simulink library "packLibrary"  (R2022b)
settings: Solver=VariableStepAuto  StartTime=0.0  StopTime=10.0  RelTol=1e-3
undefined symbols (not defined in the file): battery_builder_rtmsupport, gcbh
libraries: packLibrary_lib x12
settings Model: Creator=DELL  LastModifiedBy=DELL

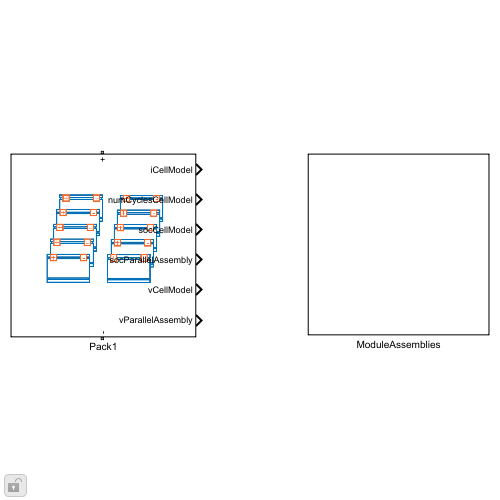
[thumbnail: Simulink's stored preview of the top-level diagram]
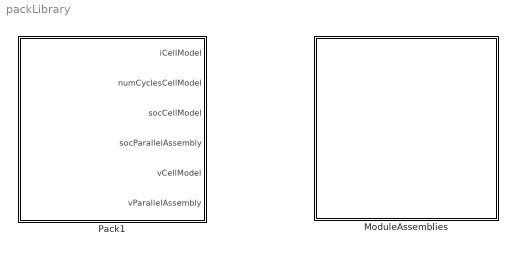
== system packLibrary ==
  ModuleAssemblies : Subsystem
  Pack1 : Subsystem  LoadFcn=battery_builder_rtmsupport('loadfcn',gcbh);
      settings: CopyFcn=battery_builder_rtmsupport('copyfcn',gcbh);  PreCopyFcn=battery_builder_rtmsupport('precopyfcn',gcbh);  PreDeleteFcn=battery_builder_rtmsupport('predeletefcn',gcbh);  PortSchema="{\"entries\":[{\"content\":{\"sides\":[{\"content\":{\"connectorIds\":[\"LConn1\"]},\"type\":\"ConnectorPlacement.EquallySpacedRectSide\",\"uuid\":\"28c6eb33-4d49-4fb1-9cde-b9dfdd77c876\"},{\"content\":{\"connectorIds\":[\"RConn1\"],\"side\":\"RIGHT\"},\"type\":\"ConnectorPlacement.EquallySpacedRectSide\",\"uuid\":\"b9810162-5634-4adf-aff8-c39045d02da2\"},{\"content\":{\"connectorIds\":[],\"side\":\"TOP\"},\"type\":\"ConnectorPlacement.EquallySpacedRectSide\",\"uuid\":\"1ba0f325-5e56-4337-925f-22d4ca88eb4a\"},{\"content\":{\"connectorIds\":[\"Out1\",\"Out2\",\"Out3\",\"Out4\",\"Out5\",\"Out6\"],\"side\":\"BOTTOM\"},\"type\":\"ConnectorPlacement.EquallySpacedRectSide\",\"uuid\":\"96c4fc69-b9f6-473b-8733-ab7f3394c566\"}]},\"type\":\"ConnectorPlacement.EquallySpacedConnector\",\"uuid\":\"e67f4e04-d31b-4901-b860-df486ab909d4\"}],\"packageUris\":[\"http://schema.mathworks.com/mf0/Connector/R2020b\"],\"version\":\"1.0\"}"
      mask Display: image('$imagefile')

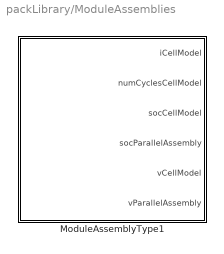
== system packLibrary/ModuleAssemblies ==
  ModuleAssemblyType1 : Subsystem  LoadFcn=battery_builder_rtmsupport('loadfcn',gcbh);
      settings: CopyFcn=battery_builder_rtmsupport('copyfcn',gcbh);  PreCopyFcn=battery_builder_rtmsupport('precopyfcn',gcbh);  PreDeleteFcn=battery_builder_rtmsupport('predeletefcn',gcbh);  PortSchema="{\"entries\":[{\"content\":{\"sides\":[{\"content\":{\"connectorIds\":[\"LConn1\"]},\"type\":\"ConnectorPlacement.EquallySpacedRectSide\",\"uuid\":\"28c6eb33-4d49-4fb1-9cde-b9dfdd77c876\"},{\"content\":{\"connectorIds\":[\"RConn1\"],\"side\":\"RIGHT\"},\"type\":\"ConnectorPlacement.EquallySpacedRectSide\",\"uuid\":\"b9810162-5634-4adf-aff8-c39045d02da2\"},{\"content\":{\"connectorIds\":[],\"side\":\"TOP\"},\"type\":\"ConnectorPlacement.EquallySpacedRectSide\",\"uuid\":\"1ba0f325-5e56-4337-925f-22d4ca88eb4a\"},{\"content\":{\"connectorIds\":[\"Out1\",\"Out2\",\"Out3\",\"Out4\",\"Out5\",\"Out6\"],\"side\":\"BOTTOM\"},\"type\":\"ConnectorPlacement.EquallySpacedRectSide\",\"uuid\":\"d11a51c6-486f-4741-a229-6ae1ae8804c6\"}]},\"type\":\"ConnectorPlacement.EquallySpacedConnector\",\"uuid\":\"e67f4e04-d31b-4901-b860-df486ab909d4\"}],\"packageUris\":[\"http://schema.mathworks.com/mf0/Connector/R2020b\"],\"version\":\"1.0\"}"
      mask Display: image('$imagefile')

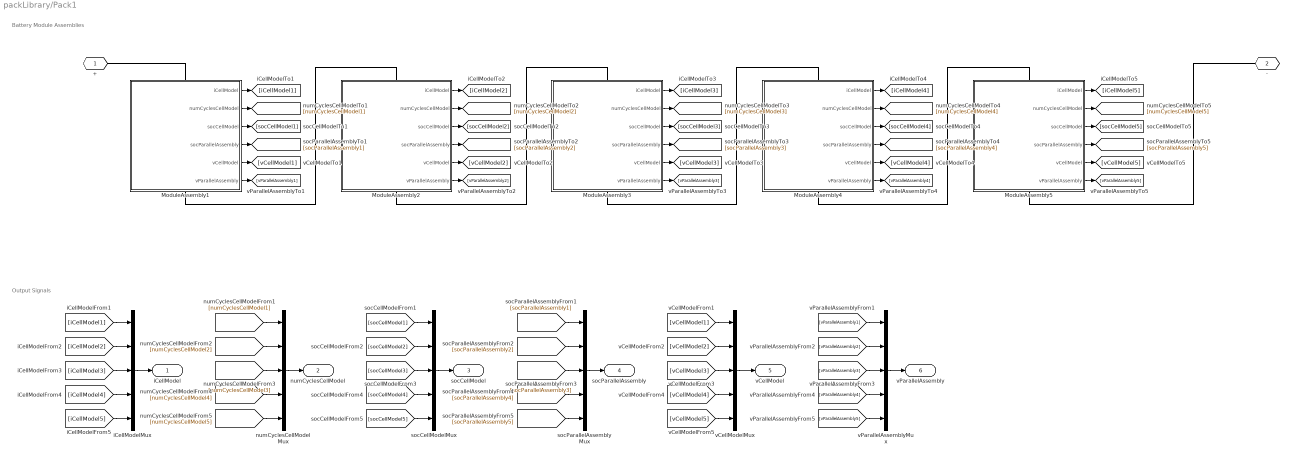
== system packLibrary/Pack1 ==
  note: Battery Module Assemblies
  note: Output Signals
  ModuleAssembly1 : Subsystem  LoadFcn=battery_builder_rtmsupport('loadfcn',gcbh);
      settings: CopyFcn=battery_builder_rtmsupport('copyfcn',gcbh);  PreCopyFcn=battery_builder_rtmsupport('precopyfcn',gcbh);  PreDeleteFcn=battery_builder_rtmsupport('predeletefcn',gcbh);  PortSchema="{\"entries\":[{\"content\":{\"sides\":[{\"content\":{\"connectorIds\":[\"LConn1\"]},\"type\":\"ConnectorPlacement.EquallySpacedRectSide\",\"uuid\":\"28c6eb33-4d49-4fb1-9cde-b9dfdd77c876\"},{\"content\":{\"connectorIds\":[\"RConn1\"],\"side\":\"RIGHT\"},\"type\":\"ConnectorPlacement.EquallySpacedRectSide\",\"uuid\":\"b9810162-5634-4adf-aff8-c39045d02da2\"},{\"content\":{\"connectorIds\":[],\"side\":\"TOP\"},\"type\":\"ConnectorPlacement.EquallySpacedRectSide\",\"uuid\":\"1ba0f325-5e56-4337-925f-22d4ca88eb4a\"},{\"content\":{\"connectorIds\":[\"Out1\",\"Out2\",\"Out3\",\"Out4\",\"Out5\",\"Out6\"],\"side\":\"BOTTOM\"},\"type\":\"ConnectorPlacement.EquallySpacedRectSide\",\"uuid\":\"d11a51c6-486f-4741-a229-6ae1ae8804c6\"}]},\"type\":\"ConnectorPlacement.EquallySpacedConnector\",\"uuid\":\"e67f4e04-d31b-4901-b860-df486ab909d4\"}],\"packageUris\":[\"http://schema.mathworks.com/mf0/Connector/R2020b\"],\"version\":\"1.0\"}"
      mask Display: image('$imagefile')
  ModuleAssembly2 : Subsystem  LoadFcn=battery_builder_rtmsupport('loadfcn',gcbh);
      settings: CopyFcn=battery_builder_rtmsupport('copyfcn',gcbh);  PreCopyFcn=battery_builder_rtmsupport('precopyfcn',gcbh);  PreDeleteFcn=battery_builder_rtmsupport('predeletefcn',gcbh);  PortSchema="{\"entries\":[{\"content\":{\"sides\":[{\"content\":{\"connectorIds\":[\"LConn1\"]},\"type\":\"ConnectorPlacement.EquallySpacedRectSide\",\"uuid\":\"28c6eb33-4d49-4fb1-9cde-b9dfdd77c876\"},{\"content\":{\"connectorIds\":[\"RConn1\"],\"side\":\"RIGHT\"},\"type\":\"ConnectorPlacement.EquallySpacedRectSide\",\"uuid\":\"b9810162-5634-4adf-aff8-c39045d02da2\"},{\"content\":{\"connectorIds\":[],\"side\":\"TOP\"},\"type\":\"ConnectorPlacement.EquallySpacedRectSide\",\"uuid\":\"1ba0f325-5e56-4337-925f-22d4ca88eb4a\"},{\"content\":{\"connectorIds\":[\"Out1\",\"Out2\",\"Out3\",\"Out4\",\"Out5\",\"Out6\"],\"side\":\"BOTTOM\"},\"type\":\"ConnectorPlacement.EquallySpacedRectSide\",\"uuid\":\"d11a51c6-486f-4741-a229-6ae1ae8804c6\"}]},\"type\":\"ConnectorPlacement.EquallySpacedConnector\",\"uuid\":\"e67f4e04-d31b-4901-b860-df486ab909d4\"}],\"packageUris\":[\"http://schema.mathworks.com/mf0/Connector/R2020b\"],\"version\":\"1.0\"}"
      mask Display: image('$imagefile')
  ModuleAssembly3 : Subsystem  LoadFcn=battery_builder_rtmsupport('loadfcn',gcbh);
      settings: CopyFcn=battery_builder_rtmsupport('copyfcn',gcbh);  PreCopyFcn=battery_builder_rtmsupport('precopyfcn',gcbh);  PreDeleteFcn=battery_builder_rtmsupport('predeletefcn',gcbh);  PortSchema="{\"entries\":[{\"content\":{\"sides\":[{\"content\":{\"connectorIds\":[\"LConn1\"]},\"type\":\"ConnectorPlacement.EquallySpacedRectSide\",\"uuid\":\"28c6eb33-4d49-4fb1-9cde-b9dfdd77c876\"},{\"content\":{\"connectorIds\":[\"RConn1\"],\"side\":\"RIGHT\"},\"type\":\"ConnectorPlacement.EquallySpacedRectSide\",\"uuid\":\"b9810162-5634-4adf-aff8-c39045d02da2\"},{\"content\":{\"connectorIds\":[],\"side\":\"TOP\"},\"type\":\"ConnectorPlacement.EquallySpacedRectSide\",\"uuid\":\"1ba0f325-5e56-4337-925f-22d4ca88eb4a\"},{\"content\":{\"connectorIds\":[\"Out1\",\"Out2\",\"Out3\",\"Out4\",\"Out5\",\"Out6\"],\"side\":\"BOTTOM\"},\"type\":\"ConnectorPlacement.EquallySpacedRectSide\",\"uuid\":\"d11a51c6-486f-4741-a229-6ae1ae8804c6\"}]},\"type\":\"ConnectorPlacement.EquallySpacedConnector\",\"uuid\":\"e67f4e04-d31b-4901-b860-df486ab909d4\"}],\"packageUris\":[\"http://schema.mathworks.com/mf0/Connector/R2020b\"],\"version\":\"1.0\"}"
      mask Display: image('$imagefile')
  ModuleAssembly4 : Subsystem  LoadFcn=battery_builder_rtmsupport('loadfcn',gcbh);
      settings: CopyFcn=battery_builder_rtmsupport('copyfcn',gcbh);  PreCopyFcn=battery_builder_rtmsupport('precopyfcn',gcbh);  PreDeleteFcn=battery_builder_rtmsupport('predeletefcn',gcbh);  PortSchema="{\"entries\":[{\"content\":{\"sides\":[{\"content\":{\"connectorIds\":[\"LConn1\"]},\"type\":\"ConnectorPlacement.EquallySpacedRectSide\",\"uuid\":\"28c6eb33-4d49-4fb1-9cde-b9dfdd77c876\"},{\"content\":{\"connectorIds\":[\"RConn1\"],\"side\":\"RIGHT\"},\"type\":\"ConnectorPlacement.EquallySpacedRectSide\",\"uuid\":\"b9810162-5634-4adf-aff8-c39045d02da2\"},{\"content\":{\"connectorIds\":[],\"side\":\"TOP\"},\"type\":\"ConnectorPlacement.EquallySpacedRectSide\",\"uuid\":\"1ba0f325-5e56-4337-925f-22d4ca88eb4a\"},{\"content\":{\"connectorIds\":[\"Out1\",\"Out2\",\"Out3\",\"Out4\",\"Out5\",\"Out6\"],\"side\":\"BOTTOM\"},\"type\":\"ConnectorPlacement.EquallySpacedRectSide\",\"uuid\":\"d11a51c6-486f-4741-a229-6ae1ae8804c6\"}]},\"type\":\"ConnectorPlacement.EquallySpacedConnector\",\"uuid\":\"e67f4e04-d31b-4901-b860-df486ab909d4\"}],\"packageUris\":[\"http://schema.mathworks.com/mf0/Connector/R2020b\"],\"version\":\"1.0\"}"
      mask Display: image('$imagefile')
  ModuleAssembly5 : Subsystem  LoadFcn=battery_builder_rtmsupport('loadfcn',gcbh);
      settings: CopyFcn=battery_builder_rtmsupport('copyfcn',gcbh);  PreCopyFcn=battery_builder_rtmsupport('precopyfcn',gcbh);  PreDeleteFcn=battery_builder_rtmsupport('predeletefcn',gcbh);  PortSchema="{\"entries\":[{\"content\":{\"sides\":[{\"content\":{\"connectorIds\":[\"LConn1\"]},\"type\":\"ConnectorPlacement.EquallySpacedRectSide\",\"uuid\":\"28c6eb33-4d49-4fb1-9cde-b9dfdd77c876\"},{\"content\":{\"connectorIds\":[\"RConn1\"],\"side\":\"RIGHT\"},\"type\":\"ConnectorPlacement.EquallySpacedRectSide\",\"uuid\":\"b9810162-5634-4adf-aff8-c39045d02da2\"},{\"content\":{\"connectorIds\":[],\"side\":\"TOP\"},\"type\":\"ConnectorPlacement.EquallySpacedRectSide\",\"uuid\":\"1ba0f325-5e56-4337-925f-22d4ca88eb4a\"},{\"content\":{\"connectorIds\":[\"Out1\",\"Out2\",\"Out3\",\"Out4\",\"Out5\",\"Out6\"],\"side\":\"BOTTOM\"},\"type\":\"ConnectorPlacement.EquallySpacedRectSide\",\"uuid\":\"d11a51c6-486f-4741-a229-6ae1ae8804c6\"}]},\"type\":\"ConnectorPlacement.EquallySpacedConnector\",\"uuid\":\"e67f4e04-d31b-4901-b860-df486ab909d4\"}],\"packageUris\":[\"http://schema.mathworks.com/mf0/Connector/R2020b\"],\"version\":\"1.0\"}"
      mask Display: image('$imagefile')
  iCellModelMux : Mux  Inputs=5
  numCyclesCellModelMux : Mux  Inputs=5
  socCellModelMux : Mux  Inputs=5
  socParallelAssemblyMux : Mux  Inputs=5
  vCellModelMux : Mux  Inputs=5
  vParallelAssemblyMux : Mux  Inputs=5
  + : PMIOPort  Side=Left
  - : PMIOPort  Port=2  Side=Right
  iCellModel : Outport
  numCyclesCellModel : Outport  Port=2
  socCellModel : Outport  Port=3
  socParallelAssembly : Outport  Port=4
  vCellModel : Outport  Port=5
  vParallelAssembly : Outport  Port=6
  wires:
  ModuleAssembly1/1(iCellModel) -> [iCellModel1]
  iCellModelMux/1 -> iCellModel/1
  [iCellModel1] -> iCellModelMux/1
  ModuleAssembly1/2(numCyclesCellModel) -> [numCyclesCellModel1]
  numCyclesCellModelMux/1 -> numCyclesCellModel/1
  [numCyclesCellModel1] -> numCyclesCellModelMux/1
  ModuleAssembly1/3(socCellModel) -> [socCellModel1]
  socCellModelMux/1 -> socCellModel/1
  [socCellModel1] -> socCellModelMux/1
  ModuleAssembly1/4(socParallelAssembly) -> [socParallelAssembly1]
  socParallelAssemblyMux/1 -> socParallelAssembly/1
  [socParallelAssembly1] -> socParallelAssemblyMux/1
  ModuleAssembly1/5(vCellModel) -> [vCellModel1]
  vCellModelMux/1 -> vCellModel/1
  [vCellModel1] -> vCellModelMux/1
  ModuleAssembly1/6(vParallelAssembly) -> [vParallelAssembly1]
  vParallelAssemblyMux/1 -> vParallelAssembly/1
  [vParallelAssembly1] -> vParallelAssemblyMux/1
  ModuleAssembly2/1(iCellModel) -> [iCellModel2]
  [iCellModel2] -> iCellModelMux/2
  ModuleAssembly2/2(numCyclesCellModel) -> [numCyclesCellModel2]
  [numCyclesCellModel2] -> numCyclesCellModelMux/2
  ModuleAssembly2/3(socCellModel) -> [socCellModel2]
  [socCellModel2] -> socCellModelMux/2
  ModuleAssembly2/4(socParallelAssembly) -> [socParallelAssembly2]
  [socParallelAssembly2] -> socParallelAssemblyMux/2
  ModuleAssembly2/5(vCellModel) -> [vCellModel2]
  [vCellModel2] -> vCellModelMux/2
  ModuleAssembly2/6(vParallelAssembly) -> [vParallelAssembly2]
  [vParallelAssembly2] -> vParallelAssemblyMux/2
  ModuleAssembly3/1(iCellModel) -> [iCellModel3]
  [iCellModel3] -> iCellModelMux/3
  ModuleAssembly3/2(numCyclesCellModel) -> [numCyclesCellModel3]
  [numCyclesCellModel3] -> numCyclesCellModelMux/3
  ModuleAssembly3/3(socCellModel) -> [socCellModel3]
  [socCellModel3] -> socCellModelMux/3
  ModuleAssembly3/4(socParallelAssembly) -> [socParallelAssembly3]
  [socParallelAssembly3] -> socParallelAssemblyMux/3
  ModuleAssembly3/5(vCellModel) -> [vCellModel3]
  [vCellModel3] -> vCellModelMux/3
  ModuleAssembly3/6(vParallelAssembly) -> [vParallelAssembly3]
  [vParallelAssembly3] -> vParallelAssemblyMux/3
  ModuleAssembly4/1(iCellModel) -> [iCellModel4]
  [iCellModel4] -> iCellModelMux/4
  ModuleAssembly4/2(numCyclesCellModel) -> [numCyclesCellModel4]
  [numCyclesCellModel4] -> numCyclesCellModelMux/4
  ModuleAssembly4/3(socCellModel) -> [socCellModel4]
  [socCellModel4] -> socCellModelMux/4
  ModuleAssembly4/4(socParallelAssembly) -> [socParallelAssembly4]
  [socParallelAssembly4] -> socParallelAssemblyMux/4
  ModuleAssembly4/5(vCellModel) -> [vCellModel4]
  [vCellModel4] -> vCellModelMux/4
  ModuleAssembly4/6(vParallelAssembly) -> [vParallelAssembly4]
  [vParallelAssembly4] -> vParallelAssemblyMux/4
  ModuleAssembly5/1(iCellModel) -> [iCellModel5]
  [iCellModel5] -> iCellModelMux/5
  ModuleAssembly5/2(numCyclesCellModel) -> [numCyclesCellModel5]
  [numCyclesCellModel5] -> numCyclesCellModelMux/5
  ModuleAssembly5/3(socCellModel) -> [socCellModel5]
  [socCellModel5] -> socCellModelMux/5
  ModuleAssembly5/4(socParallelAssembly) -> [socParallelAssembly5]
  [socParallelAssembly5] -> socParallelAssemblyMux/5
  ModuleAssembly5/5(vCellModel) -> [vCellModel5]
  [vCellModel5] -> vCellModelMux/5
  ModuleAssembly5/6(vParallelAssembly) -> [vParallelAssembly5]
  [vParallelAssembly5] -> vParallelAssemblyMux/5
  connections:
  ModuleAssembly2/LConn1 -- ModuleAssembly1/RConn1
  ModuleAssembly3/LConn1 -- ModuleAssembly2/RConn1
  ModuleAssembly4/LConn1 -- ModuleAssembly3/RConn1
  ModuleAssembly5/LConn1 -- ModuleAssembly4/RConn1
  ModuleAssembly1/LConn1 -- +/RConn1
  ModuleAssembly5/RConn1 -- -/RConn1

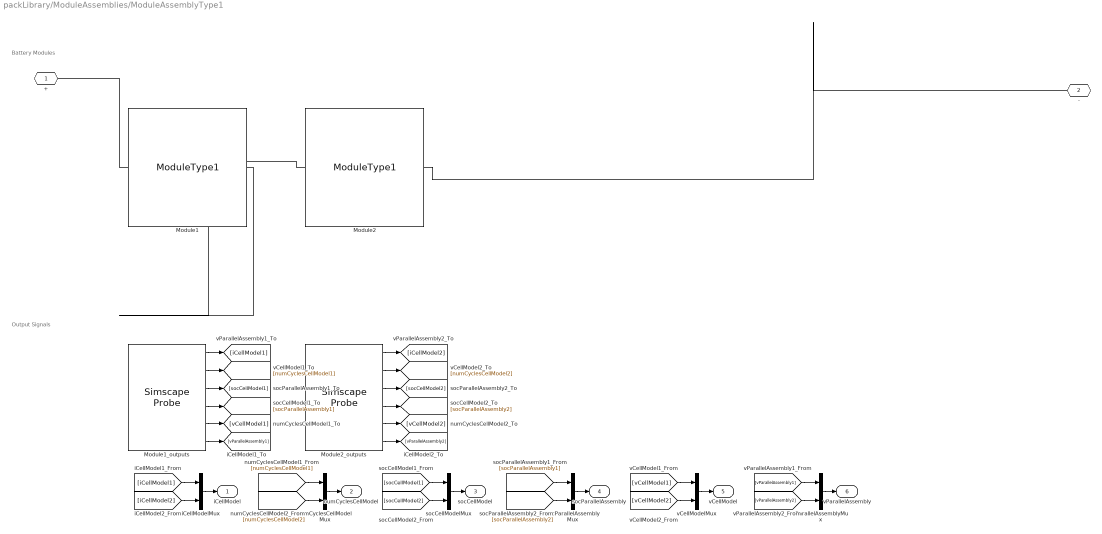
== system packLibrary/ModuleAssemblies/ModuleAssemblyType1 ==
  note: Battery Modules
  note: Output Signals
  Module1 : packLibrary_lib/Modules/ModuleType1  SOC_vec=[0, .1, .25, .5, .75, .9, 1]  V0_vec=[3.5057, 3.566, 3.6337, 3.7127, 3.9259, 4.0777, 4.1928] V  V_range=[0, inf] V  R0_vec=[.0085, .0085, .0087, .0082, .0083, .0085, .0085] Ohm  AH=27 A*hr  extrapolation_option=simscape.enum.extrapolation.nearest  P=3  S=11  iCellModel_specify=off  iCellModel_priority=None  iCellModel=0 A  iCellModel_nominal_specify=off  iCellModel_nominal_unit=A  iCellModel_nominal_value=1  vCellModel_specify=off  vCellModel_priority=None  vCellModel=0 V  vCellModel_nominal_specify=off  vCellModel_nominal_unit=V  vCellModel_nominal_value=1  socCellModel_specify=off  socCellModel_priority=High  socCellModel=1  socCellModel_nominal_specify=off  socCellModel_nominal_unit=1  socCellModel_nominal_value=1  numCyclesCellModel_specify=off  numCyclesCellModel_priority=High  numCyclesCellModel=0  numCyclesCellModel_nominal_specify=off  numCyclesCellModel_nominal_unit=1  numCyclesCellModel_nominal_value=1  vParallelAssembly_specify=off  vParallelAssembly_priority=None  vParallelAssembly=repmat(0, 11, 1) V  vParallelAssembly_nominal_specify=off  vParallelAssembly_nominal_unit=V  vParallelAssembly_nominal_value=1  socParallelAssembly_specify=off  socParallelAssembly_priority=None  socParallelAssembly=repmat(1, 11, 1)  socParallelAssembly_nominal_specify=off  socParallelAssembly_nominal_unit=1  socParallelAssembly_nominal_value=1
      settings: InternalSimscapePortConfiguration="{\"Bottom\":[{\"id\":\"n\",\"label\":\"-\",\"type\":\"foundation.electrical.electrical\"}],\"Left\":[],\"Right\":[],\"Top\":[{\"id\":\"p\",\"label\":\"+\",\"type\":\"foundation.electrical.electrical\"}]}"
  Module1_outputs : SimscapeProbe  BoundBlock=3  Variables={iCellModel, numCyclesCellModel, socCellModel, socParallelAssembly, vCellModel, vParallelAssembly}
  Module2 : packLibrary_lib/Modules/ModuleType1  SOC_vec=[0, .1, .25, .5, .75, .9, 1]  V0_vec=[3.5057, 3.566, 3.6337, 3.7127, 3.9259, 4.0777, 4.1928] V  V_range=[0, inf] V  R0_vec=[.0085, .0085, .0087, .0082, .0083, .0085, .0085] Ohm  AH=27 A*hr  extrapolation_option=simscape.enum.extrapolation.nearest  P=3  S=11  iCellModel_specify=off  iCellModel_priority=None  iCellModel=0 A  iCellModel_nominal_specify=off  iCellModel_nominal_unit=A  iCellModel_nominal_value=1  vCellModel_specify=off  vCellModel_priority=None  vCellModel=0 V  vCellModel_nominal_specify=off  vCellModel_nominal_unit=V  vCellModel_nominal_value=1  socCellModel_specify=off  socCellModel_priority=High  socCellModel=1  socCellModel_nominal_specify=off  socCellModel_nominal_unit=1  socCellModel_nominal_value=1  numCyclesCellModel_specify=off  numCyclesCellModel_priority=High  numCyclesCellModel=0  numCyclesCellModel_nominal_specify=off  numCyclesCellModel_nominal_unit=1  numCyclesCellModel_nominal_value=1  vParallelAssembly_specify=off  vParallelAssembly_priority=None  vParallelAssembly=repmat(0, 11, 1) V  vParallelAssembly_nominal_specify=off  vParallelAssembly_nominal_unit=V  vParallelAssembly_nominal_value=1  socParallelAssembly_specify=off  socParallelAssembly_priority=None  socParallelAssembly=repmat(1, 11, 1)  socParallelAssembly_nominal_specify=off  socParallelAssembly_nominal_unit=1  socParallelAssembly_nominal_value=1
      settings: InternalSimscapePortConfiguration="{\"Bottom\":[{\"id\":\"n\",\"label\":\"-\",\"type\":\"foundation.electrical.electrical\"}],\"Left\":[],\"Right\":[],\"Top\":[{\"id\":\"p\",\"label\":\"+\",\"type\":\"foundation.electrical.electrical\"}]}"
  Module2_outputs : SimscapeProbe  BoundBlock=4  Variables={iCellModel, numCyclesCellModel, socCellModel, socParallelAssembly, vCellModel, vParallelAssembly}
  iCellModelMux : Mux  Inputs=2
  numCyclesCellModelMux : Mux  Inputs=2
  socCellModelMux : Mux  Inputs=2
  socParallelAssemblyMux : Mux  Inputs=2
  vCellModelMux : Mux  Inputs=2
  vParallelAssemblyMux : Mux  Inputs=2
  + : PMIOPort  Side=Left
  - : PMIOPort  Port=2  Side=Right
  iCellModel : Outport
  numCyclesCellModel : Outport  Port=2
  socCellModel : Outport  Port=3
  socParallelAssembly : Outport  Port=4
  vCellModel : Outport  Port=5
  vParallelAssembly : Outport  Port=6
  wires:
  Module1_outputs/6 -> [vParallelAssembly1]
  iCellModelMux/1 -> iCellModel/1
  [iCellModel1] -> iCellModelMux/1
  Module1_outputs/5 -> [vCellModel1]
  numCyclesCellModelMux/1 -> numCyclesCellModel/1
  [numCyclesCellModel1] -> numCyclesCellModelMux/1
  Module1_outputs/4 -> [socParallelAssembly1]
  socCellModelMux/1 -> socCellModel/1
  [socCellModel1] -> socCellModelMux/1
  Module1_outputs/3 -> [socCellModel1]
  socParallelAssemblyMux/1 -> socParallelAssembly/1
  [socParallelAssembly1] -> socParallelAssemblyMux/1
  Module1_outputs/2 -> [numCyclesCellModel1]
  vCellModelMux/1 -> vCellModel/1
  [vCellModel1] -> vCellModelMux/1
  Module1_outputs/1 -> [iCellModel1]
  vParallelAssemblyMux/1 -> vParallelAssembly/1
  [vParallelAssembly1] -> vParallelAssemblyMux/1
  Module2_outputs/6 -> [vParallelAssembly2]
  [iCellModel2] -> iCellModelMux/2
  Module2_outputs/5 -> [vCellModel2]
  [numCyclesCellModel2] -> numCyclesCellModelMux/2
  Module2_outputs/4 -> [socParallelAssembly2]
  [socCellModel2] -> socCellModelMux/2
  Module2_outputs/3 -> [socCellModel2]
  [socParallelAssembly2] -> socParallelAssemblyMux/2
  Module2_outputs/2 -> [numCyclesCellModel2]
  [vCellModel2] -> vCellModelMux/2
  Module2_outputs/1 -> [iCellModel2]
  [vParallelAssembly2] -> vParallelAssemblyMux/2
  connections:
  Module2/LConn1 -- Module1/RConn1
  Module1/LConn1 -- +/RConn1
  Module2/RConn1 -- -/RConn1

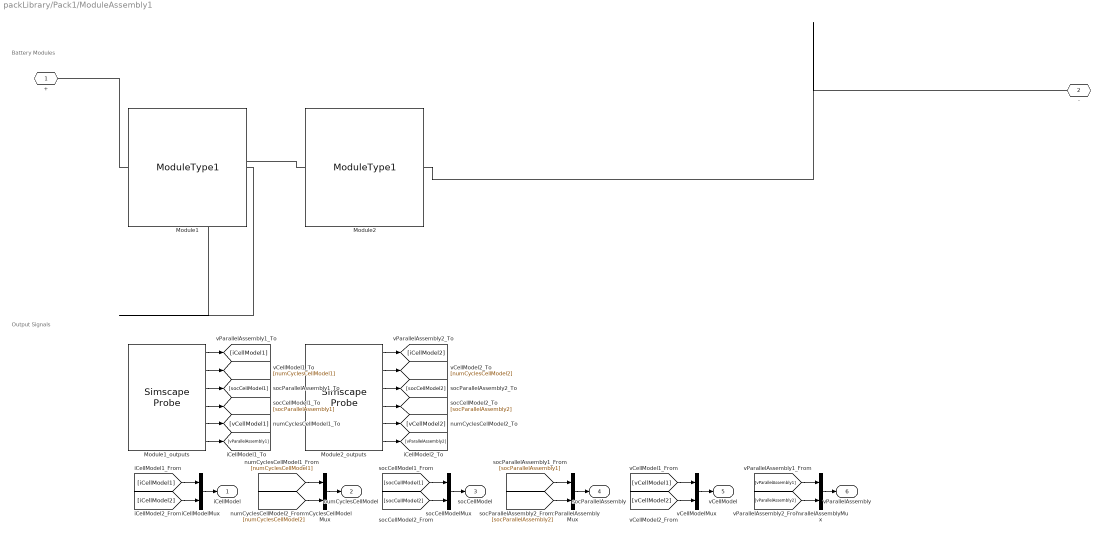
== system packLibrary/Pack1/ModuleAssembly1 ==
  note: Output Signals
  note: Battery Modules
  Module1 : packLibrary_lib/Modules/ModuleType1  SOC_vec=[0, .1, .25, .5, .75, .9, 1]  V0_vec=[3.5057, 3.566, 3.6337, 3.7127, 3.9259, 4.0777, 4.1928] V  V_range=[0, inf] V  R0_vec=[.0085, .0085, .0087, .0082, .0083, .0085, .0085] Ohm  AH=27 A*hr  extrapolation_option=simscape.enum.extrapolation.nearest  P=3  S=11  iCellModel_specify=off  iCellModel_priority=None  iCellModel=0 A  iCellModel_nominal_specify=off  iCellModel_nominal_unit=A  iCellModel_nominal_value=1  vCellModel_specify=off  vCellModel_priority=None  vCellModel=0 V  vCellModel_nominal_specify=off  vCellModel_nominal_unit=V  vCellModel_nominal_value=1  socCellModel_specify=off  socCellModel_priority=High  socCellModel=1  socCellModel_nominal_specify=off  socCellModel_nominal_unit=1  socCellModel_nominal_value=1  numCyclesCellModel_specify=off  numCyclesCellModel_priority=High  numCyclesCellModel=0  numCyclesCellModel_nominal_specify=off  numCyclesCellModel_nominal_unit=1  numCyclesCellModel_nominal_value=1  vParallelAssembly_specify=off  vParallelAssembly_priority=None  vParallelAssembly=repmat(0, 11, 1) V  vParallelAssembly_nominal_specify=off  vParallelAssembly_nominal_unit=V  vParallelAssembly_nominal_value=1  socParallelAssembly_specify=off  socParallelAssembly_priority=None  socParallelAssembly=repmat(1, 11, 1)  socParallelAssembly_nominal_specify=off  socParallelAssembly_nominal_unit=1  socParallelAssembly_nominal_value=1
      settings: InternalSimscapePortConfiguration="{\"Bottom\":[{\"id\":\"n\",\"label\":\"-\",\"type\":\"foundation.electrical.electrical\"}],\"Left\":[],\"Right\":[],\"Top\":[{\"id\":\"p\",\"label\":\"+\",\"type\":\"foundation.electrical.electrical\"}]}"
  Module1_outputs : SimscapeProbe  BoundBlock=49  Variables={iCellModel, numCyclesCellModel, socCellModel, socParallelAssembly, vCellModel, vParallelAssembly}
  Module2 : packLibrary_lib/Modules/ModuleType1  SOC_vec=[0, .1, .25, .5, .75, .9, 1]  V0_vec=[3.5057, 3.566, 3.6337, 3.7127, 3.9259, 4.0777, 4.1928] V  V_range=[0, inf] V  R0_vec=[.0085, .0085, .0087, .0082, .0083, .0085, .0085] Ohm  AH=27 A*hr  extrapolation_option=simscape.enum.extrapolation.nearest  P=3  S=11  iCellModel_specify=off  iCellModel_priority=None  iCellModel=0 A  iCellModel_nominal_specify=off  iCellModel_nominal_unit=A  iCellModel_nominal_value=1  vCellModel_specify=off  vCellModel_priority=None  vCellModel=0 V  vCellModel_nominal_specify=off  vCellModel_nominal_unit=V  vCellModel_nominal_value=1  socCellModel_specify=off  socCellModel_priority=High  socCellModel=1  socCellModel_nominal_specify=off  socCellModel_nominal_unit=1  socCellModel_nominal_value=1  numCyclesCellModel_specify=off  numCyclesCellModel_priority=High  numCyclesCellModel=0  numCyclesCellModel_nominal_specify=off  numCyclesCellModel_nominal_unit=1  numCyclesCellModel_nominal_value=1  vParallelAssembly_specify=off  vParallelAssembly_priority=None  vParallelAssembly=repmat(0, 11, 1) V  vParallelAssembly_nominal_specify=off  vParallelAssembly_nominal_unit=V  vParallelAssembly_nominal_value=1  socParallelAssembly_specify=off  socParallelAssembly_priority=None  socParallelAssembly=repmat(1, 11, 1)  socParallelAssembly_nominal_specify=off  socParallelAssembly_nominal_unit=1  socParallelAssembly_nominal_value=1
      settings: InternalSimscapePortConfiguration="{\"Bottom\":[{\"id\":\"n\",\"label\":\"-\",\"type\":\"foundation.electrical.electrical\"}],\"Left\":[],\"Right\":[],\"Top\":[{\"id\":\"p\",\"label\":\"+\",\"type\":\"foundation.electrical.electrical\"}]}"
  Module2_outputs : SimscapeProbe  BoundBlock=51  Variables={iCellModel, numCyclesCellModel, socCellModel, socParallelAssembly, vCellModel, vParallelAssembly}
  iCellModelMux : Mux  Inputs=2
  numCyclesCellModelMux : Mux  Inputs=2
  socCellModelMux : Mux  Inputs=2
  socParallelAssemblyMux : Mux  Inputs=2
  vCellModelMux : Mux  Inputs=2
  vParallelAssemblyMux : Mux  Inputs=2
  + : PMIOPort  Side=Left
  - : PMIOPort  Port=2  Side=Right
  iCellModel : Outport
  numCyclesCellModel : Outport  Port=2
  socCellModel : Outport  Port=3
  socParallelAssembly : Outport  Port=4
  vCellModel : Outport  Port=5
  vParallelAssembly : Outport  Port=6
  wires:
  [vParallelAssembly2] -> vParallelAssemblyMux/2
  Module2_outputs/1 -> [iCellModel2]
  [vCellModel2] -> vCellModelMux/2
  Module2_outputs/2 -> [numCyclesCellModel2]
  [socParallelAssembly2] -> socParallelAssemblyMux/2
  Module2_outputs/3 -> [socCellModel2]
  [socCellModel2] -> socCellModelMux/2
  Module2_outputs/4 -> [socParallelAssembly2]
  [numCyclesCellModel2] -> numCyclesCellModelMux/2
  Module2_outputs/5 -> [vCellModel2]
  [iCellModel2] -> iCellModelMux/2
  Module2_outputs/6 -> [vParallelAssembly2]
  [vParallelAssembly1] -> vParallelAssemblyMux/1
  vParallelAssemblyMux/1 -> vParallelAssembly/1
  Module1_outputs/1 -> [iCellModel1]
  [vCellModel1] -> vCellModelMux/1
  vCellModelMux/1 -> vCellModel/1
  Module1_outputs/2 -> [numCyclesCellModel1]
  [socParallelAssembly1] -> socParallelAssemblyMux/1
  socParallelAssemblyMux/1 -> socParallelAssembly/1
  Module1_outputs/3 -> [socCellModel1]
  [socCellModel1] -> socCellModelMux/1
  socCellModelMux/1 -> socCellModel/1
  Module1_outputs/4 -> [socParallelAssembly1]
  [numCyclesCellModel1] -> numCyclesCellModelMux/1
  numCyclesCellModelMux/1 -> numCyclesCellModel/1
  Module1_outputs/5 -> [vCellModel1]
  [iCellModel1] -> iCellModelMux/1
  iCellModelMux/1 -> iCellModel/1
  Module1_outputs/6 -> [vParallelAssembly1]
  connections:
  Module2/RConn1 -- -/RConn1
  Module1/LConn1 -- +/RConn1
  Module2/LConn1 -- Module1/RConn1

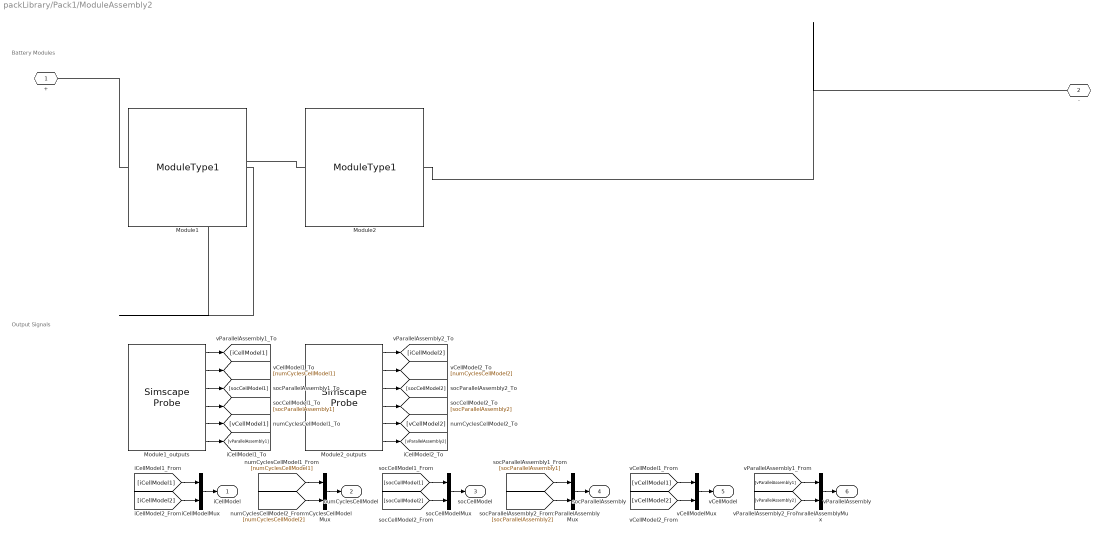
== system packLibrary/Pack1/ModuleAssembly2 ==
  note: Output Signals
  note: Battery Modules
  Module1 : packLibrary_lib/Modules/ModuleType1  SOC_vec=[0, .1, .25, .5, .75, .9, 1]  V0_vec=[3.5057, 3.566, 3.6337, 3.7127, 3.9259, 4.0777, 4.1928] V  V_range=[0, inf] V  R0_vec=[.0085, .0085, .0087, .0082, .0083, .0085, .0085] Ohm  AH=27 A*hr  extrapolation_option=simscape.enum.extrapolation.nearest  P=3  S=11  iCellModel_specify=off  iCellModel_priority=None  iCellModel=0 A  iCellModel_nominal_specify=off  iCellModel_nominal_unit=A  iCellModel_nominal_value=1  vCellModel_specify=off  vCellModel_priority=None  vCellModel=0 V  vCellModel_nominal_specify=off  vCellModel_nominal_unit=V  vCellModel_nominal_value=1  socCellModel_specify=off  socCellModel_priority=High  socCellModel=1  socCellModel_nominal_specify=off  socCellModel_nominal_unit=1  socCellModel_nominal_value=1  numCyclesCellModel_specify=off  numCyclesCellModel_priority=High  numCyclesCellModel=0  numCyclesCellModel_nominal_specify=off  numCyclesCellModel_nominal_unit=1  numCyclesCellModel_nominal_value=1  vParallelAssembly_specify=off  vParallelAssembly_priority=None  vParallelAssembly=repmat(0, 11, 1) V  vParallelAssembly_nominal_specify=off  vParallelAssembly_nominal_unit=V  vParallelAssembly_nominal_value=1  socParallelAssembly_specify=off  socParallelAssembly_priority=None  socParallelAssembly=repmat(1, 11, 1)  socParallelAssembly_nominal_specify=off  socParallelAssembly_nominal_unit=1  socParallelAssembly_nominal_value=1
      settings: InternalSimscapePortConfiguration="{\"Bottom\":[{\"id\":\"n\",\"label\":\"-\",\"type\":\"foundation.electrical.electrical\"}],\"Left\":[],\"Right\":[],\"Top\":[{\"id\":\"p\",\"label\":\"+\",\"type\":\"foundation.electrical.electrical\"}]}"
  Module1_outputs : SimscapeProbe  BoundBlock=94  Variables={iCellModel, numCyclesCellModel, socCellModel, socParallelAssembly, vCellModel, vParallelAssembly}
  Module2 : packLibrary_lib/Modules/ModuleType1  SOC_vec=[0, .1, .25, .5, .75, .9, 1]  V0_vec=[3.5057, 3.566, 3.6337, 3.7127, 3.9259, 4.0777, 4.1928] V  V_range=[0, inf] V  R0_vec=[.0085, .0085, .0087, .0082, .0083, .0085, .0085] Ohm  AH=27 A*hr  extrapolation_option=simscape.enum.extrapolation.nearest  P=3  S=11  iCellModel_specify=off  iCellModel_priority=None  iCellModel=0 A  iCellModel_nominal_specify=off  iCellModel_nominal_unit=A  iCellModel_nominal_value=1  vCellModel_specify=off  vCellModel_priority=None  vCellModel=0 V  vCellModel_nominal_specify=off  vCellModel_nominal_unit=V  vCellModel_nominal_value=1  socCellModel_specify=off  socCellModel_priority=High  socCellModel=1  socCellModel_nominal_specify=off  socCellModel_nominal_unit=1  socCellModel_nominal_value=1  numCyclesCellModel_specify=off  numCyclesCellModel_priority=High  numCyclesCellModel=0  numCyclesCellModel_nominal_specify=off  numCyclesCellModel_nominal_unit=1  numCyclesCellModel_nominal_value=1  vParallelAssembly_specify=off  vParallelAssembly_priority=None  vParallelAssembly=repmat(0, 11, 1) V  vParallelAssembly_nominal_specify=off  vParallelAssembly_nominal_unit=V  vParallelAssembly_nominal_value=1  socParallelAssembly_specify=off  socParallelAssembly_priority=None  socParallelAssembly=repmat(1, 11, 1)  socParallelAssembly_nominal_specify=off  socParallelAssembly_nominal_unit=1  socParallelAssembly_nominal_value=1
      settings: InternalSimscapePortConfiguration="{\"Bottom\":[{\"id\":\"n\",\"label\":\"-\",\"type\":\"foundation.electrical.electrical\"}],\"Left\":[],\"Right\":[],\"Top\":[{\"id\":\"p\",\"label\":\"+\",\"type\":\"foundation.electrical.electrical\"}]}"
  Module2_outputs : SimscapeProbe  BoundBlock=96  Variables={iCellModel, numCyclesCellModel, socCellModel, socParallelAssembly, vCellModel, vParallelAssembly}
  iCellModelMux : Mux  Inputs=2
  numCyclesCellModelMux : Mux  Inputs=2
  socCellModelMux : Mux  Inputs=2
  socParallelAssemblyMux : Mux  Inputs=2
  vCellModelMux : Mux  Inputs=2
  vParallelAssemblyMux : Mux  Inputs=2
  + : PMIOPort  Side=Left
  - : PMIOPort  Port=2  Side=Right
  iCellModel : Outport
  numCyclesCellModel : Outport  Port=2
  socCellModel : Outport  Port=3
  socParallelAssembly : Outport  Port=4
  vCellModel : Outport  Port=5
  vParallelAssembly : Outport  Port=6
  wires:
  [vParallelAssembly2] -> vParallelAssemblyMux/2
  Module2_outputs/1 -> [iCellModel2]
  [vCellModel2] -> vCellModelMux/2
  Module2_outputs/2 -> [numCyclesCellModel2]
  [socParallelAssembly2] -> socParallelAssemblyMux/2
  Module2_outputs/3 -> [socCellModel2]
  [socCellModel2] -> socCellModelMux/2
  Module2_outputs/4 -> [socParallelAssembly2]
  [numCyclesCellModel2] -> numCyclesCellModelMux/2
  Module2_outputs/5 -> [vCellModel2]
  [iCellModel2] -> iCellModelMux/2
  Module2_outputs/6 -> [vParallelAssembly2]
  [vParallelAssembly1] -> vParallelAssemblyMux/1
  vParallelAssemblyMux/1 -> vParallelAssembly/1
  Module1_outputs/1 -> [iCellModel1]
  [vCellModel1] -> vCellModelMux/1
  vCellModelMux/1 -> vCellModel/1
  Module1_outputs/2 -> [numCyclesCellModel1]
  [socParallelAssembly1] -> socParallelAssemblyMux/1
  socParallelAssemblyMux/1 -> socParallelAssembly/1
  Module1_outputs/3 -> [socCellModel1]
  [socCellModel1] -> socCellModelMux/1
  socCellModelMux/1 -> socCellModel/1
  Module1_outputs/4 -> [socParallelAssembly1]
  [numCyclesCellModel1] -> numCyclesCellModelMux/1
  numCyclesCellModelMux/1 -> numCyclesCellModel/1
  Module1_outputs/5 -> [vCellModel1]
  [iCellModel1] -> iCellModelMux/1
  iCellModelMux/1 -> iCellModel/1
  Module1_outputs/6 -> [vParallelAssembly1]
  connections:
  Module2/RConn1 -- -/RConn1
  Module1/LConn1 -- +/RConn1
  Module2/LConn1 -- Module1/RConn1

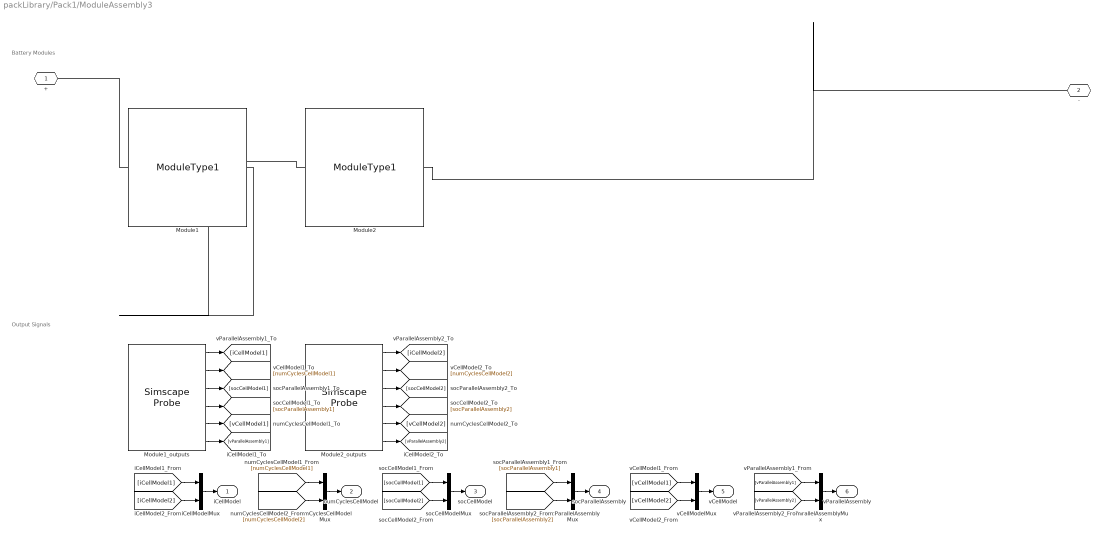
== system packLibrary/Pack1/ModuleAssembly3 ==
  note: Output Signals
  note: Battery Modules
  Module1 : packLibrary_lib/Modules/ModuleType1  SOC_vec=[0, .1, .25, .5, .75, .9, 1]  V0_vec=[3.5057, 3.566, 3.6337, 3.7127, 3.9259, 4.0777, 4.1928] V  V_range=[0, inf] V  R0_vec=[.0085, .0085, .0087, .0082, .0083, .0085, .0085] Ohm  AH=27 A*hr  extrapolation_option=simscape.enum.extrapolation.nearest  P=3  S=11  iCellModel_specify=off  iCellModel_priority=None  iCellModel=0 A  iCellModel_nominal_specify=off  iCellModel_nominal_unit=A  iCellModel_nominal_value=1  vCellModel_specify=off  vCellModel_priority=None  vCellModel=0 V  vCellModel_nominal_specify=off  vCellModel_nominal_unit=V  vCellModel_nominal_value=1  socCellModel_specify=off  socCellModel_priority=High  socCellModel=1  socCellModel_nominal_specify=off  socCellModel_nominal_unit=1  socCellModel_nominal_value=1  numCyclesCellModel_specify=off  numCyclesCellModel_priority=High  numCyclesCellModel=0  numCyclesCellModel_nominal_specify=off  numCyclesCellModel_nominal_unit=1  numCyclesCellModel_nominal_value=1  vParallelAssembly_specify=off  vParallelAssembly_priority=None  vParallelAssembly=repmat(0, 11, 1) V  vParallelAssembly_nominal_specify=off  vParallelAssembly_nominal_unit=V  vParallelAssembly_nominal_value=1  socParallelAssembly_specify=off  socParallelAssembly_priority=None  socParallelAssembly=repmat(1, 11, 1)  socParallelAssembly_nominal_specify=off  socParallelAssembly_nominal_unit=1  socParallelAssembly_nominal_value=1
      settings: InternalSimscapePortConfiguration="{\"Bottom\":[{\"id\":\"n\",\"label\":\"-\",\"type\":\"foundation.electrical.electrical\"}],\"Left\":[],\"Right\":[],\"Top\":[{\"id\":\"p\",\"label\":\"+\",\"type\":\"foundation.electrical.electrical\"}]}"
  Module1_outputs : SimscapeProbe  BoundBlock=139  Variables={iCellModel, numCyclesCellModel, socCellModel, socParallelAssembly, vCellModel, vParallelAssembly}
  Module2 : packLibrary_lib/Modules/ModuleType1  SOC_vec=[0, .1, .25, .5, .75, .9, 1]  V0_vec=[3.5057, 3.566, 3.6337, 3.7127, 3.9259, 4.0777, 4.1928] V  V_range=[0, inf] V  R0_vec=[.0085, .0085, .0087, .0082, .0083, .0085, .0085] Ohm  AH=27 A*hr  extrapolation_option=simscape.enum.extrapolation.nearest  P=3  S=11  iCellModel_specify=off  iCellModel_priority=None  iCellModel=0 A  iCellModel_nominal_specify=off  iCellModel_nominal_unit=A  iCellModel_nominal_value=1  vCellModel_specify=off  vCellModel_priority=None  vCellModel=0 V  vCellModel_nominal_specify=off  vCellModel_nominal_unit=V  vCellModel_nominal_value=1  socCellModel_specify=off  socCellModel_priority=High  socCellModel=1  socCellModel_nominal_specify=off  socCellModel_nominal_unit=1  socCellModel_nominal_value=1  numCyclesCellModel_specify=off  numCyclesCellModel_priority=High  numCyclesCellModel=0  numCyclesCellModel_nominal_specify=off  numCyclesCellModel_nominal_unit=1  numCyclesCellModel_nominal_value=1  vParallelAssembly_specify=off  vParallelAssembly_priority=None  vParallelAssembly=repmat(0, 11, 1) V  vParallelAssembly_nominal_specify=off  vParallelAssembly_nominal_unit=V  vParallelAssembly_nominal_value=1  socParallelAssembly_specify=off  socParallelAssembly_priority=None  socParallelAssembly=repmat(1, 11, 1)  socParallelAssembly_nominal_specify=off  socParallelAssembly_nominal_unit=1  socParallelAssembly_nominal_value=1
      settings: InternalSimscapePortConfiguration="{\"Bottom\":[{\"id\":\"n\",\"label\":\"-\",\"type\":\"foundation.electrical.electrical\"}],\"Left\":[],\"Right\":[],\"Top\":[{\"id\":\"p\",\"label\":\"+\",\"type\":\"foundation.electrical.electrical\"}]}"
  Module2_outputs : SimscapeProbe  BoundBlock=141  Variables={iCellModel, numCyclesCellModel, socCellModel, socParallelAssembly, vCellModel, vParallelAssembly}
  iCellModelMux : Mux  Inputs=2
  numCyclesCellModelMux : Mux  Inputs=2
  socCellModelMux : Mux  Inputs=2
  socParallelAssemblyMux : Mux  Inputs=2
  vCellModelMux : Mux  Inputs=2
  vParallelAssemblyMux : Mux  Inputs=2
  + : PMIOPort  Side=Left
  - : PMIOPort  Port=2  Side=Right
  iCellModel : Outport
  numCyclesCellModel : Outport  Port=2
  socCellModel : Outport  Port=3
  socParallelAssembly : Outport  Port=4
  vCellModel : Outport  Port=5
  vParallelAssembly : Outport  Port=6
  wires:
  [vParallelAssembly2] -> vParallelAssemblyMux/2
  Module2_outputs/1 -> [iCellModel2]
  [vCellModel2] -> vCellModelMux/2
  Module2_outputs/2 -> [numCyclesCellModel2]
  [socParallelAssembly2] -> socParallelAssemblyMux/2
  Module2_outputs/3 -> [socCellModel2]
  [socCellModel2] -> socCellModelMux/2
  Module2_outputs/4 -> [socParallelAssembly2]
  [numCyclesCellModel2] -> numCyclesCellModelMux/2
  Module2_outputs/5 -> [vCellModel2]
  [iCellModel2] -> iCellModelMux/2
  Module2_outputs/6 -> [vParallelAssembly2]
  [vParallelAssembly1] -> vParallelAssemblyMux/1
  vParallelAssemblyMux/1 -> vParallelAssembly/1
  Module1_outputs/1 -> [iCellModel1]
  [vCellModel1] -> vCellModelMux/1
  vCellModelMux/1 -> vCellModel/1
  Module1_outputs/2 -> [numCyclesCellModel1]
  [socParallelAssembly1] -> socParallelAssemblyMux/1
  socParallelAssemblyMux/1 -> socParallelAssembly/1
  Module1_outputs/3 -> [socCellModel1]
  [socCellModel1] -> socCellModelMux/1
  socCellModelMux/1 -> socCellModel/1
  Module1_outputs/4 -> [socParallelAssembly1]
  [numCyclesCellModel1] -> numCyclesCellModelMux/1
  numCyclesCellModelMux/1 -> numCyclesCellModel/1
  Module1_outputs/5 -> [vCellModel1]
  [iCellModel1] -> iCellModelMux/1
  iCellModelMux/1 -> iCellModel/1
  Module1_outputs/6 -> [vParallelAssembly1]
  connections:
  Module2/RConn1 -- -/RConn1
  Module1/LConn1 -- +/RConn1
  Module2/LConn1 -- Module1/RConn1

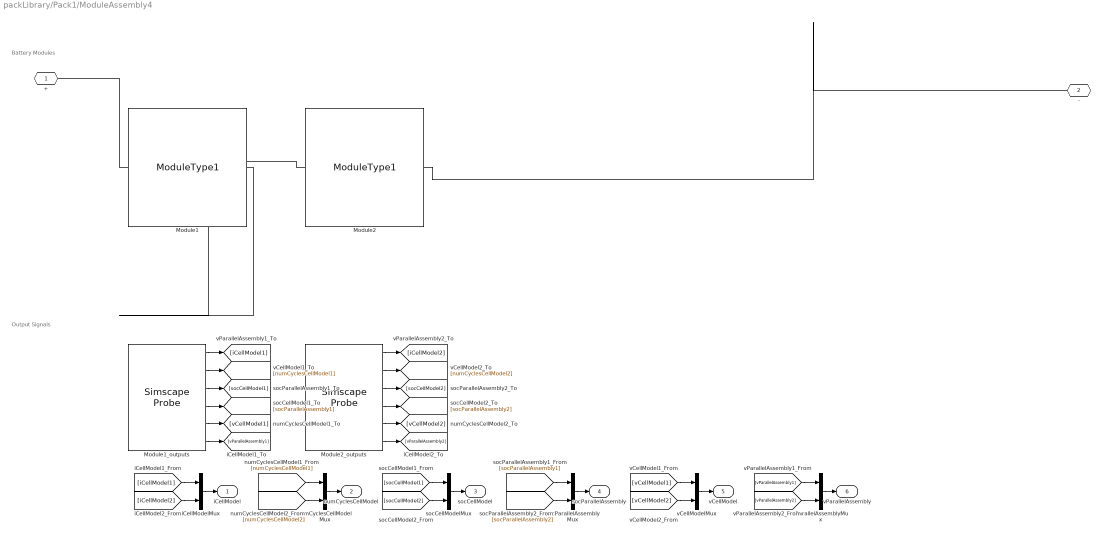
== system packLibrary/Pack1/ModuleAssembly4 ==
  note: Output Signals
  note: Battery Modules
  Module1 : packLibrary_lib/Modules/ModuleType1  SOC_vec=[0, .1, .25, .5, .75, .9, 1]  V0_vec=[3.5057, 3.566, 3.6337, 3.7127, 3.9259, 4.0777, 4.1928] V  V_range=[0, inf] V  R0_vec=[.0085, .0085, .0087, .0082, .0083, .0085, .0085] Ohm  AH=27 A*hr  extrapolation_option=simscape.enum.extrapolation.nearest  P=3  S=11  iCellModel_specify=off  iCellModel_priority=None  iCellModel=0 A  iCellModel_nominal_specify=off  iCellModel_nominal_unit=A  iCellModel_nominal_value=1  vCellModel_specify=off  vCellModel_priority=None  vCellModel=0 V  vCellModel_nominal_specify=off  vCellModel_nominal_unit=V  vCellModel_nominal_value=1  socCellModel_specify=off  socCellModel_priority=High  socCellModel=1  socCellModel_nominal_specify=off  socCellModel_nominal_unit=1  socCellModel_nominal_value=1  numCyclesCellModel_specify=off  numCyclesCellModel_priority=High  numCyclesCellModel=0  numCyclesCellModel_nominal_specify=off  numCyclesCellModel_nominal_unit=1  numCyclesCellModel_nominal_value=1  vParallelAssembly_specify=off  vParallelAssembly_priority=None  vParallelAssembly=repmat(0, 11, 1) V  vParallelAssembly_nominal_specify=off  vParallelAssembly_nominal_unit=V  vParallelAssembly_nominal_value=1  socParallelAssembly_specify=off  socParallelAssembly_priority=None  socParallelAssembly=repmat(1, 11, 1)  socParallelAssembly_nominal_specify=off  socParallelAssembly_nominal_unit=1  socParallelAssembly_nominal_value=1
      settings: InternalSimscapePortConfiguration="{\"Bottom\":[{\"id\":\"n\",\"label\":\"-\",\"type\":\"foundation.electrical.electrical\"}],\"Left\":[],\"Right\":[],\"Top\":[{\"id\":\"p\",\"label\":\"+\",\"type\":\"foundation.electrical.electrical\"}]}"
  Module1_outputs : SimscapeProbe  BoundBlock=184  Variables={iCellModel, numCyclesCellModel, socCellModel, socParallelAssembly, vCellModel, vParallelAssembly}
  Module2 : packLibrary_lib/Modules/ModuleType1  SOC_vec=[0, .1, .25, .5, .75, .9, 1]  V0_vec=[3.5057, 3.566, 3.6337, 3.7127, 3.9259, 4.0777, 4.1928] V  V_range=[0, inf] V  R0_vec=[.0085, .0085, .0087, .0082, .0083, .0085, .0085] Ohm  AH=27 A*hr  extrapolation_option=simscape.enum.extrapolation.nearest  P=3  S=11  iCellModel_specify=off  iCellModel_priority=None  iCellModel=0 A  iCellModel_nominal_specify=off  iCellModel_nominal_unit=A  iCellModel_nominal_value=1  vCellModel_specify=off  vCellModel_priority=None  vCellModel=0 V  vCellModel_nominal_specify=off  vCellModel_nominal_unit=V  vCellModel_nominal_value=1  socCellModel_specify=off  socCellModel_priority=High  socCellModel=1  socCellModel_nominal_specify=off  socCellModel_nominal_unit=1  socCellModel_nominal_value=1  numCyclesCellModel_specify=off  numCyclesCellModel_priority=High  numCyclesCellModel=0  numCyclesCellModel_nominal_specify=off  numCyclesCellModel_nominal_unit=1  numCyclesCellModel_nominal_value=1  vParallelAssembly_specify=off  vParallelAssembly_priority=None  vParallelAssembly=repmat(0, 11, 1) V  vParallelAssembly_nominal_specify=off  vParallelAssembly_nominal_unit=V  vParallelAssembly_nominal_value=1  socParallelAssembly_specify=off  socParallelAssembly_priority=None  socParallelAssembly=repmat(1, 11, 1)  socParallelAssembly_nominal_specify=off  socParallelAssembly_nominal_unit=1  socParallelAssembly_nominal_value=1
      settings: InternalSimscapePortConfiguration="{\"Bottom\":[{\"id\":\"n\",\"label\":\"-\",\"type\":\"foundation.electrical.electrical\"}],\"Left\":[],\"Right\":[],\"Top\":[{\"id\":\"p\",\"label\":\"+\",\"type\":\"foundation.electrical.electrical\"}]}"
  Module2_outputs : SimscapeProbe  BoundBlock=186  Variables={iCellModel, numCyclesCellModel, socCellModel, socParallelAssembly, vCellModel, vParallelAssembly}
  iCellModelMux : Mux  Inputs=2
  numCyclesCellModelMux : Mux  Inputs=2
  socCellModelMux : Mux  Inputs=2
  socParallelAssemblyMux : Mux  Inputs=2
  vCellModelMux : Mux  Inputs=2
  vParallelAssemblyMux : Mux  Inputs=2
  + : PMIOPort  Side=Left
  - : PMIOPort  Port=2  Side=Right
  iCellModel : Outport
  numCyclesCellModel : Outport  Port=2
  socCellModel : Outport  Port=3
  socParallelAssembly : Outport  Port=4
  vCellModel : Outport  Port=5
  vParallelAssembly : Outport  Port=6
  wires:
  [vParallelAssembly2] -> vParallelAssemblyMux/2
  Module2_outputs/1 -> [iCellModel2]
  [vCellModel2] -> vCellModelMux/2
  Module2_outputs/2 -> [numCyclesCellModel2]
  [socParallelAssembly2] -> socParallelAssemblyMux/2
  Module2_outputs/3 -> [socCellModel2]
  [socCellModel2] -> socCellModelMux/2
  Module2_outputs/4 -> [socParallelAssembly2]
  [numCyclesCellModel2] -> numCyclesCellModelMux/2
  Module2_outputs/5 -> [vCellModel2]
  [iCellModel2] -> iCellModelMux/2
  Module2_outputs/6 -> [vParallelAssembly2]
  [vParallelAssembly1] -> vParallelAssemblyMux/1
  vParallelAssemblyMux/1 -> vParallelAssembly/1
  Module1_outputs/1 -> [iCellModel1]
  [vCellModel1] -> vCellModelMux/1
  vCellModelMux/1 -> vCellModel/1
  Module1_outputs/2 -> [numCyclesCellModel1]
  [socParallelAssembly1] -> socParallelAssemblyMux/1
  socParallelAssemblyMux/1 -> socParallelAssembly/1
  Module1_outputs/3 -> [socCellModel1]
  [socCellModel1] -> socCellModelMux/1
  socCellModelMux/1 -> socCellModel/1
  Module1_outputs/4 -> [socParallelAssembly1]
  [numCyclesCellModel1] -> numCyclesCellModelMux/1
  numCyclesCellModelMux/1 -> numCyclesCellModel/1
  Module1_outputs/5 -> [vCellModel1]
  [iCellModel1] -> iCellModelMux/1
  iCellModelMux/1 -> iCellModel/1
  Module1_outputs/6 -> [vParallelAssembly1]
  connections:
  Module2/RConn1 -- -/RConn1
  Module1/LConn1 -- +/RConn1
  Module2/LConn1 -- Module1/RConn1

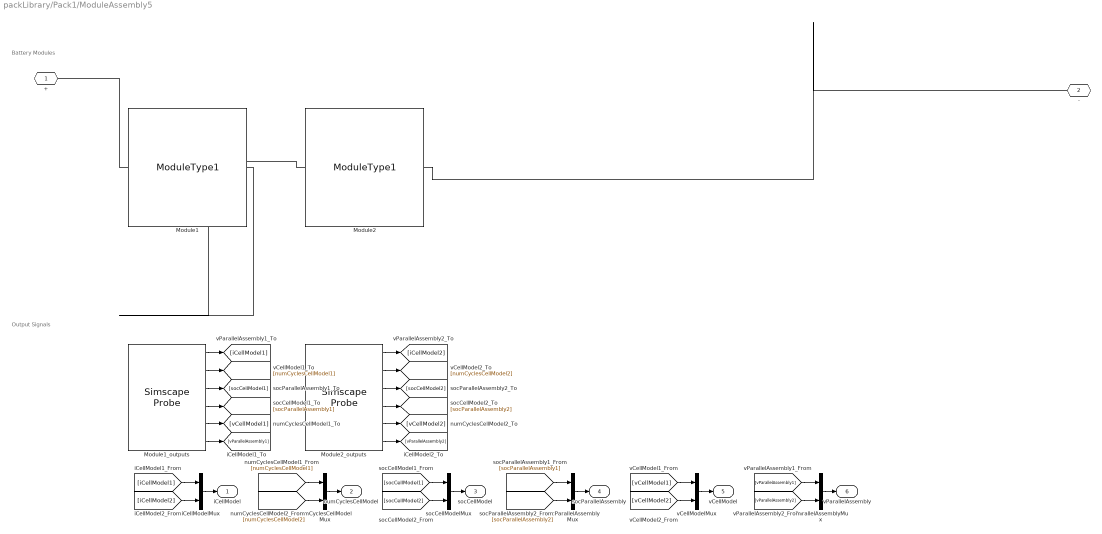
== system packLibrary/Pack1/ModuleAssembly5 ==
  note: Output Signals
  note: Battery Modules
  Module1 : packLibrary_lib/Modules/ModuleType1  SOC_vec=[0, .1, .25, .5, .75, .9, 1]  V0_vec=[3.5057, 3.566, 3.6337, 3.7127, 3.9259, 4.0777, 4.1928] V  V_range=[0, inf] V  R0_vec=[.0085, .0085, .0087, .0082, .0083, .0085, .0085] Ohm  AH=27 A*hr  extrapolation_option=simscape.enum.extrapolation.nearest  P=3  S=11  iCellModel_specify=off  iCellModel_priority=None  iCellModel=0 A  iCellModel_nominal_specify=off  iCellModel_nominal_unit=A  iCellModel_nominal_value=1  vCellModel_specify=off  vCellModel_priority=None  vCellModel=0 V  vCellModel_nominal_specify=off  vCellModel_nominal_unit=V  vCellModel_nominal_value=1  socCellModel_specify=off  socCellModel_priority=High  socCellModel=1  socCellModel_nominal_specify=off  socCellModel_nominal_unit=1  socCellModel_nominal_value=1  numCyclesCellModel_specify=off  numCyclesCellModel_priority=High  numCyclesCellModel=0  numCyclesCellModel_nominal_specify=off  numCyclesCellModel_nominal_unit=1  numCyclesCellModel_nominal_value=1  vParallelAssembly_specify=off  vParallelAssembly_priority=None  vParallelAssembly=repmat(0, 11, 1) V  vParallelAssembly_nominal_specify=off  vParallelAssembly_nominal_unit=V  vParallelAssembly_nominal_value=1  socParallelAssembly_specify=off  socParallelAssembly_priority=None  socParallelAssembly=repmat(1, 11, 1)  socParallelAssembly_nominal_specify=off  socParallelAssembly_nominal_unit=1  socParallelAssembly_nominal_value=1
      settings: InternalSimscapePortConfiguration="{\"Bottom\":[{\"id\":\"n\",\"label\":\"-\",\"type\":\"foundation.electrical.electrical\"}],\"Left\":[],\"Right\":[],\"Top\":[{\"id\":\"p\",\"label\":\"+\",\"type\":\"foundation.electrical.electrical\"}]}"
  Module1_outputs : SimscapeProbe  BoundBlock=229  Variables={iCellModel, numCyclesCellModel, socCellModel, socParallelAssembly, vCellModel, vParallelAssembly}
  Module2 : packLibrary_lib/Modules/ModuleType1  SOC_vec=[0, .1, .25, .5, .75, .9, 1]  V0_vec=[3.5057, 3.566, 3.6337, 3.7127, 3.9259, 4.0777, 4.1928] V  V_range=[0, inf] V  R0_vec=[.0085, .0085, .0087, .0082, .0083, .0085, .0085] Ohm  AH=27 A*hr  extrapolation_option=simscape.enum.extrapolation.nearest  P=3  S=11  iCellModel_specify=off  iCellModel_priority=None  iCellModel=0 A  iCellModel_nominal_specify=off  iCellModel_nominal_unit=A  iCellModel_nominal_value=1  vCellModel_specify=off  vCellModel_priority=None  vCellModel=0 V  vCellModel_nominal_specify=off  vCellModel_nominal_unit=V  vCellModel_nominal_value=1  socCellModel_specify=off  socCellModel_priority=High  socCellModel=1  socCellModel_nominal_specify=off  socCellModel_nominal_unit=1  socCellModel_nominal_value=1  numCyclesCellModel_specify=off  numCyclesCellModel_priority=High  numCyclesCellModel=0  numCyclesCellModel_nominal_specify=off  numCyclesCellModel_nominal_unit=1  numCyclesCellModel_nominal_value=1  vParallelAssembly_specify=off  vParallelAssembly_priority=None  vParallelAssembly=repmat(0, 11, 1) V  vParallelAssembly_nominal_specify=off  vParallelAssembly_nominal_unit=V  vParallelAssembly_nominal_value=1  socParallelAssembly_specify=off  socParallelAssembly_priority=None  socParallelAssembly=repmat(1, 11, 1)  socParallelAssembly_nominal_specify=off  socParallelAssembly_nominal_unit=1  socParallelAssembly_nominal_value=1
      settings: InternalSimscapePortConfiguration="{\"Bottom\":[{\"id\":\"n\",\"label\":\"-\",\"type\":\"foundation.electrical.electrical\"}],\"Left\":[],\"Right\":[],\"Top\":[{\"id\":\"p\",\"label\":\"+\",\"type\":\"foundation.electrical.electrical\"}]}"
  Module2_outputs : SimscapeProbe  BoundBlock=231  Variables={iCellModel, numCyclesCellModel, socCellModel, socParallelAssembly, vCellModel, vParallelAssembly}
  iCellModelMux : Mux  Inputs=2
  numCyclesCellModelMux : Mux  Inputs=2
  socCellModelMux : Mux  Inputs=2
  socParallelAssemblyMux : Mux  Inputs=2
  vCellModelMux : Mux  Inputs=2
  vParallelAssemblyMux : Mux  Inputs=2
  + : PMIOPort  Side=Left
  - : PMIOPort  Port=2  Side=Right
  iCellModel : Outport
  numCyclesCellModel : Outport  Port=2
  socCellModel : Outport  Port=3
  socParallelAssembly : Outport  Port=4
  vCellModel : Outport  Port=5
  vParallelAssembly : Outport  Port=6
  wires:
  [vParallelAssembly2] -> vParallelAssemblyMux/2
  Module2_outputs/1 -> [iCellModel2]
  [vCellModel2] -> vCellModelMux/2
  Module2_outputs/2 -> [numCyclesCellModel2]
  [socParallelAssembly2] -> socParallelAssemblyMux/2
  Module2_outputs/3 -> [socCellModel2]
  [socCellModel2] -> socCellModelMux/2
  Module2_outputs/4 -> [socParallelAssembly2]
  [numCyclesCellModel2] -> numCyclesCellModelMux/2
  Module2_outputs/5 -> [vCellModel2]
  [iCellModel2] -> iCellModelMux/2
  Module2_outputs/6 -> [vParallelAssembly2]
  [vParallelAssembly1] -> vParallelAssemblyMux/1
  vParallelAssemblyMux/1 -> vParallelAssembly/1
  Module1_outputs/1 -> [iCellModel1]
  [vCellModel1] -> vCellModelMux/1
  vCellModelMux/1 -> vCellModel/1
  Module1_outputs/2 -> [numCyclesCellModel1]
  [socParallelAssembly1] -> socParallelAssemblyMux/1
  socParallelAssemblyMux/1 -> socParallelAssembly/1
  Module1_outputs/3 -> [socCellModel1]
  [socCellModel1] -> socCellModelMux/1
  socCellModelMux/1 -> socCellModel/1
  Module1_outputs/4 -> [socParallelAssembly1]
  [numCyclesCellModel1] -> numCyclesCellModelMux/1
  numCyclesCellModelMux/1 -> numCyclesCellModel/1
  Module1_outputs/5 -> [vCellModel1]
  [iCellModel1] -> iCellModelMux/1
  iCellModelMux/1 -> iCellModel/1
  Module1_outputs/6 -> [vParallelAssembly1]
  connections:
  Module2/RConn1 -- -/RConn1
  Module1/LConn1 -- +/RConn1
  Module2/LConn1 -- Module1/RConn1
